simulink model "EV_X"  (Simulink 10.0)
settings: Solver=VariableStepDiscrete  StartTime=0.0  StopTime=t  RelTol=1e-3  EnableMultiTasking=on
values from neighbouring files (symbols this model uses):
  C_dc = 1/f/X_C_dc/2/pi    (= 0.00207880657305)    [debug_sim.m]    (also in sim_FFT.m = 0.000880368876163)
  C_emi = 1/f/X_C_emi/2/pi    (= 1.83329274556e-06)    [debug_sim.m]    (also in sim_FFT.m = 6.54783506897e-07)
  f = 50    [debug_sim.m]    (also in sim_FFT.m)
  fh = 0    [debug_sim.m]    (also in sim_FFT.m = supply_harmonics(i))
  Initialph_f = Initialph_f_range(k)    [debug_sim.m]    (also in sim_FFT.m = 0)
  Initialph_h = 20    [debug_sim.m]    (also in sim_FFT.m)
  L1 = X_L1/(2*pi*f)    (= 3.67999795653e-05)    [debug_sim.m]    (also in sim_FFT.m = 1.98767488989e-05)
  R1 = R1_pu*r_base    (= 0.344330909091)    [debug_sim.m]    (also in sim_FFT.m = 0.287957186544)
  R_eq = 50    [debug_sim.m]    (also in sim_FFT.m = 14.7214067278)
  T = 1e-6    (= 1e-06)    [debug_sim.m]    (also in sim_FFT.m)
  Va = supply_voltage_f(k)    [debug_sim.m]    (also in sim_FFT.m)
  Vh = 0    [debug_sim.m]    (also in sim_FFT.m = supply_voltage_h(j))
libraries: powerlib x17
settings Model: Creator=thefox  LastModifiedBy=Pascal
settings DataIOCC: LimitDataPoints=on  SignalLoggingSaveFormat=ModelDataLogs
settings OptimizationCC: ExpressionDepthLimit=2147483647
settings DebuggingCC: SolverPrmCheckMsg=warning  FcnCallInpInsideContextMsg=warning  StateNameClashWarn=warning
settings GRTTargetCC: GeneratePreprocessorConditionals=Disable all
settings ConfigComp: CovExternalEMLEnable=off

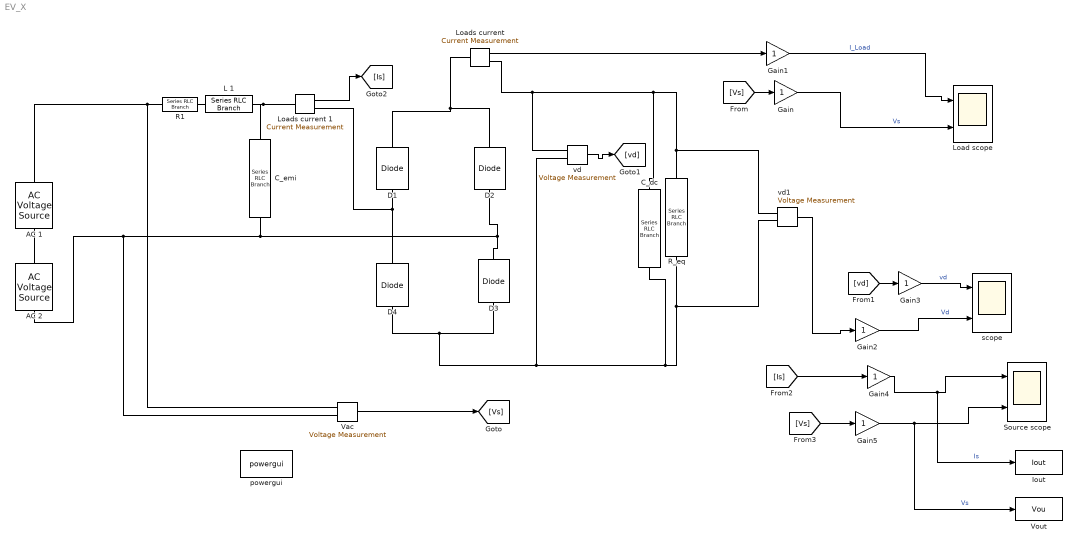
== system EV_X ==
  " scope " : Scope  NumInputPorts=2
  AC 1 : powerlib/Electrical Sources/AC Voltage Source  Amplitude=Vh  Phase=Initialph_h  Frequency=fh  SampleTime=0  Measurements=None  BusType=swing  Pref=10e3  Qref=0  Qmin=-inf  Qmax=+inf
      settings: SourceProductName=Simscape Electrical
  AC 2 : powerlib/Electrical Sources/AC Voltage Source  Amplitude=Va  Phase=Initialph_f  Frequency=f  SampleTime=0  Measurements=None  BusType=swing  Pref=10e3  Qref=0  Qmin=-inf  Qmax=+inf
      settings: SourceProductName=Simscape Electrical
  C_dc : powerlib/Elements/Series RLC Branch  LConnTagsString=__new0  RConnTagsString=__new0  BranchType=C  Resistance=10  Inductance=1e-3  SetiL0=off  InitialCurrent=0  Capacitance=C_dc  Setx0=off  InitialVoltage=0  Measurements=None
      settings: SourceProductName=Simscape Electrical
  C_emi : powerlib/Elements/Series RLC Branch  LConnTagsString=__new0  RConnTagsString=__new0  BranchType=C  Resistance=10  Inductance=1e-3  SetiL0=off  InitialCurrent=0  Capacitance=C_emi  Setx0=off  InitialVoltage=0  Measurements=None
      settings: SourceProductName=Simscape Electrical
  D{1..4} (4 alike) : powerlib/Power Electronics/Diode  Ron=0.001  Lon=0  Vf=0.8  IC=0  UseSnubber=off  Rs=500  Cs=250e-9  Measurements=off
      settings: SourceProductName=Simscape Electrical
  Gain{,1..5} (6 alike) : Gain
  Iout : ToWorkspace  VariableName=Iout  SampleTime=-1
  L 1 : powerlib/Elements/Series RLC Branch  LConnTagsString=__new0  RConnTagsString=__new0  BranchType=L  Resistance=1  Inductance=L1  SetiL0=off  InitialCurrent=0  Capacitance=1e-6  Setx0=off  InitialVoltage=0  Measurements=None
      settings: SourceProductName=Simscape Electrical
  Load scope : Scope  NumInputPorts=2
      settings: Tag=scope1
  "Loads current " : powerlib/Measurements/Current Measurement  PhasorSimulation=off  OutputType=Complex  PSBequivalent=0
      settings: SourceProductName=Simscape Electrical
  Loads current 1 : powerlib/Measurements/Current Measurement  PhasorSimulation=off  OutputType=Complex  PSBequivalent=0
      settings: SourceProductName=Simscape Electrical
  R1 : powerlib/Elements/Series RLC Branch  LConnTagsString=__new0  RConnTagsString=__new0  BranchType=R  Resistance=R1  Inductance=1e-3  SetiL0=off  InitialCurrent=0  Capacitance=1e-6  Setx0=off  InitialVoltage=0  Measurements=None
      settings: SourceProductName=Simscape Electrical
  R_eq : powerlib/Elements/Series RLC Branch  LConnTagsString=__new0  RConnTagsString=__new0  BranchType=R  Resistance=R_eq  Inductance=1e-3  SetiL0=off  InitialCurrent=0  Capacitance=1e-6  Setx0=off  InitialVoltage=0  Measurements=None
      settings: SourceProductName=Simscape Electrical
  "Source scope " : Scope  NumInputPorts=2
  Vac : powerlib/Measurements/Voltage Measurement  PhasorSimulation=off  OutputType=Complex  PSBequivalent=0
      settings: SourceProductName=Simscape Electrical
  Vout : ToWorkspace  VariableName=Vou  SampleTime=-1
  powergui : powerlib/powergui  Priority=1  SimulationMode=Discrete  SampleTime=T  frequency=60  Iterations=50  frequencyindice=50  Pbase=100e6  ErrMax=1e-4  UnitsV=kV  UnitsW=MW  buscounter=0  FunctionMessages=off  echomessages=off  EnableUseOfTLC=off  CurrentSourceSwitches=off  DisableSnubberDevices=off  DisableRonSwitches=off  DisableVfSwitches=off  DisplayEquations=off  AutomaticDiscreteSolvers=off  SolverType=Tustin/Backward Euler (TBE)  Interpol=off  ExternalGateDelay=off  methode=off  Ts=100  x0status=blocks  SPID=off  SwTol=0  HookPort=off  NonlinearTolerance=1e-4  nMaxIteration=100  ContinueOnMaxIteration=off  RestoreLinks=warning  ResistiveCurrentMeasurement=off  Frange=[0:2:500]  Ylog=off  Xlog=on  ShowGrid=off  save=off  variable=ZData  structure=S_scope  ZoomFFT=off  StartTime=0.06  cycles=2  DisplayStyle=4  fundamental=50  FreqAxis=off  MaxFrequency=1100  frequencyindicesteady=1  RmsSteady=1  display=off
      settings: SourceProductName=Simscape Electrical
  vd : powerlib/Measurements/Voltage Measurement  PhasorSimulation=off  OutputType=Complex  PSBequivalent=0
      settings: SourceProductName=Simscape Electrical
  vd1 : powerlib/Measurements/Voltage Measurement  PhasorSimulation=off  OutputType=Complex  PSBequivalent=0
      settings: SourceProductName=Simscape Electrical
  wires:
  vd/1 -> [vd]
  Vac/1 -> [Vs]
  [Vs] -> Gain/1
  Gain/1 -> Load scope/2  "Vs"
  "Loads current "/1 -> Gain1/1
  Gain1/1 -> Load scope/1  "I_Load"
  vd1/1 -> Gain2/1
  Gain2/1 -> " scope "/2  "Vd"
  [vd] -> Gain3/1
  Gain3/1 -> " scope "/1  "vd"
  Loads current 1/1 -> [Is]
  [Is] -> Gain4/1
  Gain4/1 -> "Source scope "/1, Iout/1  "Is"
  [Vs] -> Gain5/1
  Gain5/1 -> "Source scope "/2, Vout/1  "Vs"
  connections:
  D3/LConn1 -- D4/LConn1 -- vd1/LConn2 -- R_eq/LConn1 -- C_dc/LConn1 -- vd/LConn2
  D2/RConn1 -- D1/RConn1 -- "Loads current "/LConn1
  vd1/LConn1 -- R_eq/RConn1 -- C_dc/RConn1 -- "Loads current "/RConn1 -- vd/LConn1
  Loads current 1/RConn1 -- D4/RConn1 -- D1/LConn1
  R1/RConn1 -- L 1/RConn1
  L 1/LConn1 -- C_emi/RConn1 -- Loads current 1/LConn1
  C_emi/LConn1 -- Vac/LConn2 -- AC 2/LConn1 -- D3/RConn1 -- D2/LConn1
  AC 2/RConn1 -- AC 1/LConn1
  AC 1/RConn1 -- R1/LConn1 -- Vac/LConn1
